simulink model "boiler2"  (Simulink 7.8)
settings: Solver=ode45  StartTime=0.0  StopTime=100  RelTol=1e-3
settings Model: Creator=Max  LastModifiedBy=Max

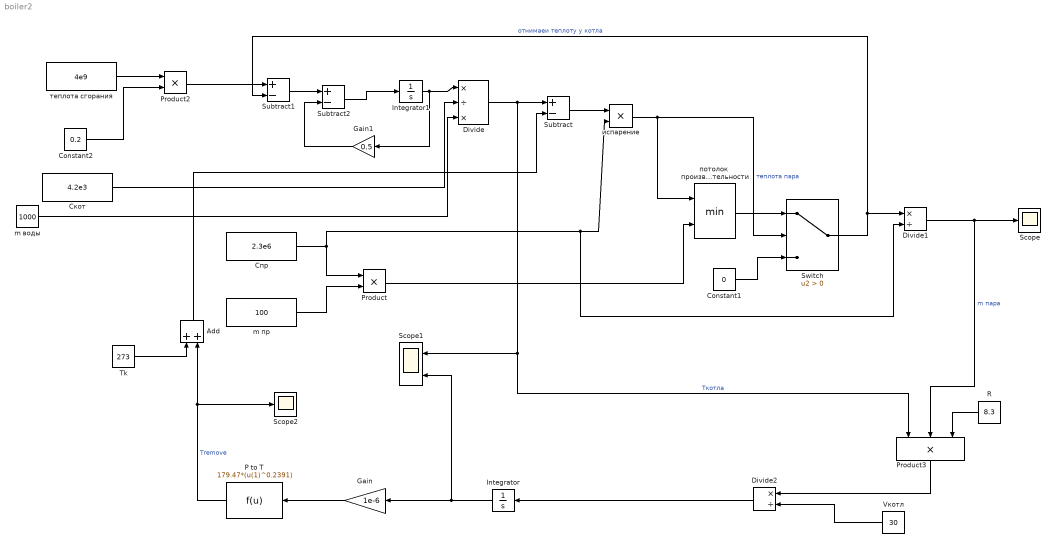
== system boiler2 ==
  Add : Sum
  Constant1 : Constant  Value=0
  Constant2 : Constant  Value=0.2
  Cкот : Constant  Value=4.2e3
  Cпр : Constant  Value=2.3e6
  Divide : Product  Inputs=*/*
  Divide1 : Product  Inputs=*/
  Divide2 : Product  Inputs=*/
  Gain : Gain  Gain=1e-6
  Gain1 : Gain  Gain=0.5
  Integrator : Integrator  InitialCondition=100000
  Integrator1 : Integrator  InitialCondition=300*4.2e6
  P to T : Fcn  Expr=179.47*(u(1)^0.2391)
  Product : Product  RndMeth=Zero
  Product2 : Product  RndMeth=Zero
  Product3 : Product  Inputs=3  RndMeth=Zero
  R : Constant  Value=8.3
  Scope : Scope
      settings: YMin=0  YMax=1.25e-007
  Scope1 : Scope  NumInputPorts=2
      settings: YMin=-5~-5  YMax=5~5
  Scope2 : Scope
      settings: YMin=0.4525  YMax=0.47  SaveName=ScopeData2
  Subtract : Sum  Inputs=+-
  Subtract1 : Sum  Inputs=+-
  Subtract2 : Sum  Inputs=+-
  Switch : Switch  Criteria=u2 > Threshold
  Tk : Constant  Value=273
  Vкотл : Constant  Value=30
  m воды : Constant  Value=1000
  m пр : Constant  Value=100
  испарение : Product  RndMeth=Zero
  потолок  производительности : MinMax  Inputs=2
  теплота сгорания : Constant  Value=4e9
  wires:
  Cпр/1 -> Product/1, испарение/2, Divide1/2
  m пр/1 -> Product/2
  Cкот/1 -> Divide/2
  Divide/1 -> Subtract/1, Scope1/1, Product3/1  "Tкотла"
  Subtract/1 -> испарение/1
  испарение/1 -> потолок  производительности/1, Switch/2  "теплота пара"
  Product/1 -> потолок  производительности/2
  Divide1/1 -> Scope/1, Product3/2  "m пара"
  потолок  производительности/1 -> Switch/1
  Switch/1 -> Divide1/1, Subtract1/2  "отнимаеи теплоту у котла"
  Constant1/1 -> Switch/3
  теплота сгорания/1 -> Product2/1
  Product2/1 -> Subtract1/1
  Constant2/1 -> Product2/2
  R/1 -> Product3/3
  Product3/1 -> Divide2/1
  Vкотл/1 -> Divide2/2
  P to T/1 -> Scope2/1, Add/2  "Tremove"
  Divide2/1 -> Integrator/1
  Integrator/1 -> Scope1/2, Gain/1
  Gain/1 -> P to T/1
  Add/1 -> Subtract/2
  Tk/1 -> Add/1
  Subtract1/1 -> Subtract2/1
  Integrator1/1 -> Divide/1, Gain1/1
  Gain1/1 -> Subtract2/2
  Subtract2/1 -> Integrator1/1
  m воды/1 -> Divide/3
